simulink model "CL_fullnonlin_prevval_ucorr"  (R2024b)
settings: Solver=VariableStepAuto  StartTime=0.0  StopTime=10.0  RelTol=1e-3
libraries: slctrl_linear x1
settings Model: Creator=kkajak  LastModifiedBy=feder
settings SolverCC: AlgebraicLoopSolver=TrustRegion
settings DataIOCC: ExternalInput=CL_long_validation_data.getElement(1)  LoadExternalInput=on  ReturnWorkspaceOutputs=off
settings DebuggingCC: UnconnectedInputMsg=warning  UnconnectedOutputMsg=warning  UnconnectedLineMsg=warning  ArithmeticOperatorsInVariantConditions=warning
settings ModelReferenceCC: EnableRefExpFcnMdlSchedulingChecks=on
settings SFSimCC: SimUseLocalCustomCode=off  CustomCodeUndefinedFunction=UseInterfaceOnly
settings RTWCC: RTWUseLocalCustomCode=off  GPUComputeCapability=3.5
settings CodeAppCC: StateflowObjectComments=on

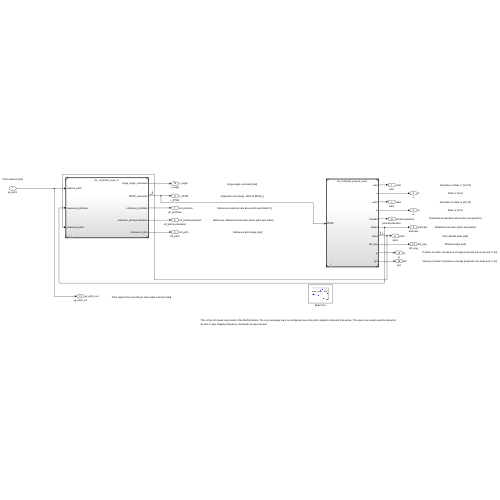
[thumbnail: Simulink's stored preview of the top-level diagram]
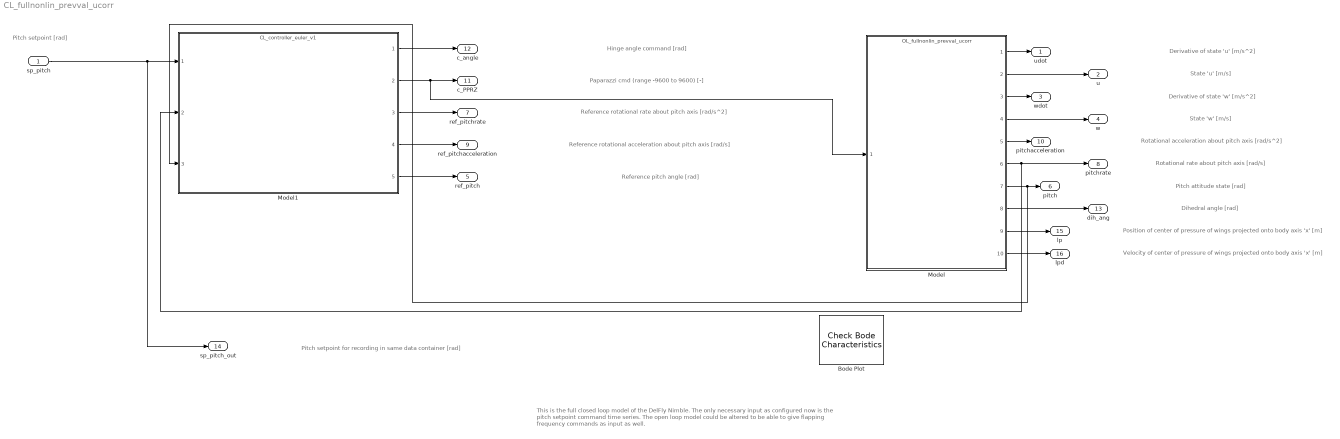
== system CL_fullnonlin_prevval_ucorr ==
  note: Pitch setpoint [rad]
  note: Pitch setpoint for recording in same data container [rad]
  note: Reference pitch angle [rad]
  note: Reference rotational acceleration about pitch axis [rad/s]
  note: Reference rotational rate about pitch axis [rad/s^2]
  note: Paparazzi cmd (range -9600 to 9600) [-]
  note: Hinge angle command [rad]
  note: Position of center of pressure of wings projected onto body axis 'x' [m]
  note: Dihedral angle [rad]
  note: Pitch attitude state [rad]
  note: Derivative of state 'u' [m/s^2]
  note: This is the full closed loop model of the DelFly Nimble. The only necessary input as configured now is the pitch setpoint command time series. The open loop model could be altered to
      | be able to give flapping frequency commands as input as well.
  note: State 'u' [m/s]
  note: Derivative of state 'w' [m/s^2]
  note: State 'w' [m/s]
  note: Rotational acceleration about pitch axis [rad/s^2]
  note: Rotational rate about pitch axis [rad/s]
  note: Velocity of center of pressure of wings projected onto body axis 'x' [m]
  sp_pitch : Inport
  Bode Plot : slctrl_linear/Check Bode  Characteristics  InstantiateOnLoad=on  SaveOperatingPoints=on  LinearizationIOs={'/Model1', 2, 'in', 'off', '';'/Model', 7, 'out', 'on', ''}  LinearizeAt=SnapshotTimes  SnapshotTimes=[0 7.9 11.9 15.9 19.9]  TriggerType=rising  SampleTime=auto  RateConversionMethod=zoh  PreWarpFreq=10  UseExactDelayModel=off  UseFullBlockNameLabels=off  UseBusSignalLabels=off  enabled=on  stopWhenAssertionFail=off  export=off  ViewDlgPos=[]  OpenViewOnLoad=off  LaunchViewOnOpen=off  FrequencyUnits=rad/s  MagnitudeUnits=dB  PhaseUnits=deg  TimeUnits=seconds  EnableUpperBound=off  UpperBoundFrequencies=[]  UpperBoundMagnitudes=[]  EnableLowerBound=off  LowerBoundFrequencies=[]  LowerBoundMagnitudes=[]
      settings: SaveToWorkspace=on  SaveName=linsys
  Model : ModelReference  ModelNameDialog=OL_fullnonlin_prevval_ucorr  SimulationMode=Normal  ModelReferenceVersion=1.73
  Model1 : ModelReference  ModelNameDialog=CL_controller_euler_v1  SimulationMode=Normal  ModelReferenceVersion=1.24
  udot : Outport  SignalName=udot
  u : Outport  Port=2  SignalName=d
  wdot : Outport  Port=3  SignalName=wdot
  w : Outport  Port=4  SignalName=w
  ref_pitch : Outport  Port=5  SignalName=ref_pitch
  pitch : Outport  Port=6  SignalName=pitch
  ref_pitchrate : Outport  Port=7  SignalName=ref_pitchrate
  pitchrate : Outport  Port=8  SignalName=pitchrate
  ref_pitchacceleration : Outport  Port=9  SignalName=ref_pitchacceleration
  pitchacceleration : Outport  Port=10  SignalName=pitchacceleration
  c_PPRZ : Outport  Port=11  SignalName=c_PPRZ
  c_angle : Outport  Port=12  SignalName=c_angle
  dih_ang : Outport  Port=13  SignalName=dih_ang
  sp_pitch_out : Outport  Port=14  SignalName=sp_pitch_out
  lp : Outport  Port=15  SignalName=lp
  lpd : Outport  Port=16  SignalName=lpd
  wires:
  Model/7 -> pitch/1, Model1/3
  Model/6 -> pitchrate/1, Model1/2
  Model/1 -> udot/1
  Model/2 -> u/1
  Model/3 -> wdot/1
  Model/4 -> w/1
  Model1/5 -> ref_pitch/1
  Model1/3 -> ref_pitchrate/1
  Model1/4 -> ref_pitchacceleration/1
  Model/5 -> pitchacceleration/1
  Model1/1 -> c_angle/1
  sp_pitch/1 -> sp_pitch_out/1, Model1/1
  Model1/2 -> c_PPRZ/1, Model/1
  Model/8 -> dih_ang/1
  Model/9 -> lp/1
  Model/10 -> lpd/1
